simulink model "INP_DRVR_test"  (R2024b)
settings: Solver=VariableStepAuto  StartTime=0.0  StopTime=10.0  RelTol=1e-3
libraries: simulink x1, INP_DRVR x1
settings Model: Creator=blatak  LastModifiedBy=blatak

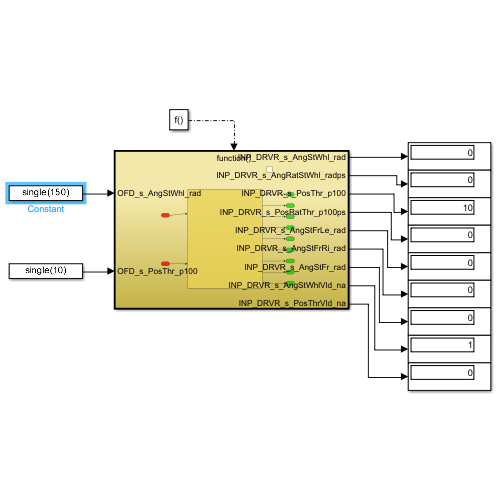
[thumbnail: Simulink's stored preview of the top-level diagram]
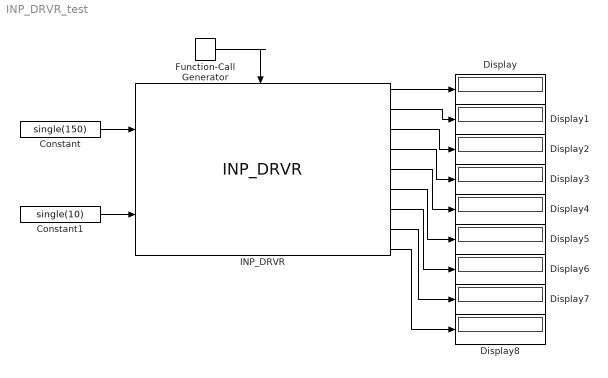
== system INP_DRVR_test ==
  Constant : Constant  Value=single(150)
  Constant1 : Constant  Value=single(10)
  Display{,1..8} (9 alike) : Display
  Function-Call Generator : simulink/Ports & Subsystems/Function-Call Generator  sample_time=0.005  numberOfIterations=1  DisallowWideOutput=off
  INP_DRVR : INP_DRVR/INP_DRVR  Description=Driver actuation processing  SystemSampleTime=-1  VariantActivationTime=update diagram  AllowFlexibleInterface=on  Latency=0  AutoFrameSizeCalculation=off
  wires:
  Function-Call Generator/1 -> INP_DRVR/Trigger
  Constant/1 -> INP_DRVR/1
  Constant1/1 -> INP_DRVR/2
  INP_DRVR/1 -> Display/1
  INP_DRVR/2 -> Display1/1
  INP_DRVR/3 -> Display2/1
  INP_DRVR/4 -> Display3/1
  INP_DRVR/5 -> Display4/1
  INP_DRVR/6 -> Display5/1
  INP_DRVR/7 -> Display6/1
  INP_DRVR/8 -> Display7/1
  INP_DRVR/9 -> Display8/1
